simulink model "Sano"  (R2024b)
settings: Solver=ode15s  StartTime=0.0  StopTime=30.0  MaxStep=1E-3  RelTol=1e-3
libraries: slpidlib x1
settings Model: Creator=leslie  LastModifiedBy=leslie
settings DataIOCC: ReturnWorkspaceOutputs=off  TimeSaveName=t
settings DebuggingCC: AlgebraicLoopMsg=none  ArtificialAlgebraicLoopMsg=none  MaxConsecutiveZCsMsg=none  InheritedTsInSrcMsg=none  MultiTaskCondExecSysMsg=none  UnknownTsInhSupMsg=none  OperatingPointInterfaceChecksumMismatchMsg=none

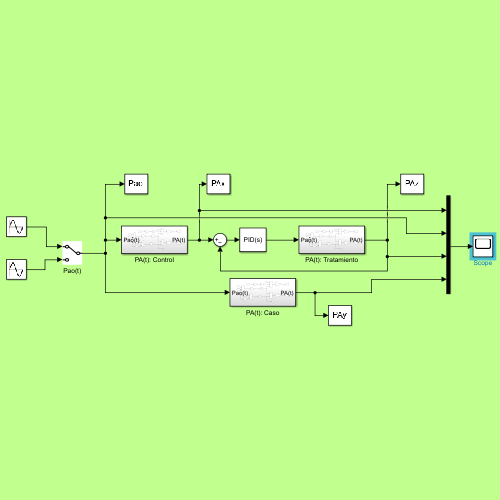
[thumbnail: Simulink's stored preview of the top-level diagram]
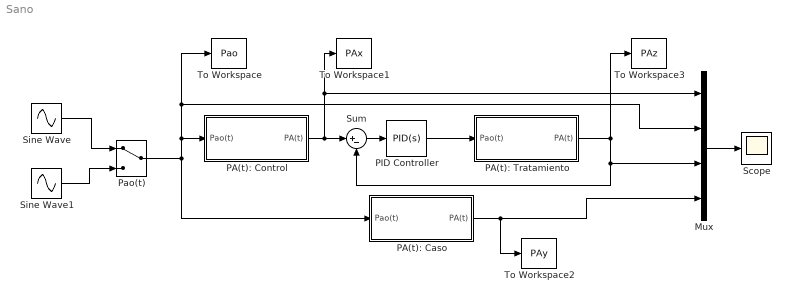
== system Sano ==
  Mux : Mux
  PA(t): Caso : Subsystem
  PA(t): Control : Subsystem
  PA(t): Tratamiento : Subsystem
  PID Controller : slpidlib/PID Controller  Controller=PID  Form=Parallel  TimeDomain=Continuous-time  UseExternalTs=off  SampleTime=-1  IntegratorMethod=Forward Euler  FilterMethod=Forward Euler  ControllerParametersSource=internal  P=15.8953606940144  I=452.120770004536  UseKiTs=off  D=0.0428965162903509  UseExternalDerivativeSource=off  N=198.651405283432  UseFilter=on  TunerSelectOption=Transfer Function Based (PID Tuner App)  InitialConditionSource=internal  InitialConditionForIntegrator=0  InitialConditionForFilter=0  DifferentiatorICPrevScaledInput=0  ExternalReset=none  TrackingMode=off  Kt=1  LimitOutput=off  SatLimitsSource=internal  UpperSaturationLimit=inf  LowerSaturationLimit=-inf  LinearizeAsGain=on  AntiWindupMode=none  Kb=1  LimitIntegrator=off  UpperIntegratorSaturationLimit=inf  LowerIntegratorSaturationLimit=-inf  POutMin=[]  POutMax=[]  IOutMin=[]  IOutMax=[]  DOutMin=[]  DOutMax=[]  NOutMin=[]  NOutMax=[]  SumOutMin=[]  SumOutMax=[]  SaturationOutMin=[]  SaturationOutMax=[]  PParamMin=[]  PParamMax=[]  IParamMin=[]  IParamMax=[]  DParamMin=[]  DParamMax=[]  NParamMin=[]  NParamMax=[]  KbParamMin=[]  KbParamMax=[]  KtParamMin=[]  KtParamMax=[]  KbOutMin=[]  KbOutMax=[]  KtOutMin=[]  KtOutMax=[]  IntegratorOutMin=[]  IntegratorOutMax=[]  FilterOutMin=[]  FilterOutMax=[]  SumI1OutMin=[]  SumI1OutMax=[]  SumI2OutMin=[]  SumI2OutMax=[]  SumI3OutMin=[]  SumI3OutMax=[]  SumI4OutMin=[]  SumI4OutMax=[]  SumDOutMin=[]  SumDOutMax=[]  DifferentiatorOutMin=[]  DifferentiatorOutMax=[]  FilterDiffOutCoefMin=[]  FilterDiffOutCoefMax=[]  ReciprocalOutMin=[]  ReciprocalOutMax=[]  SumDenOutMin=[]  SumDenOutMax=[]  SumNumOutMin=[]  SumNumOutMax=[]  DivideOutMin=[]  DivideOutMax=[]  UdiffTsProdOutMin=[]  UdiffTsProdOutMax=[]  NTsProdOutMin=[]  NTsProdOutMax=[]  UintegralTsProdOutMin=[]  UintegralTsProdOutMax=[]  UngainTsProdOutMin=[]  UngainTsProdOutMax=[]  ClampingZeroOutDataTypeStr=Inherit: Inherit via back propagation  ClampingZeroOutMin=[]  ClampingZeroOutMax=[]  FilterDenConstantOutDataTypeStr=Inherit: Inherit via back propagation  FilterDenConstantOutMin=[]  FilterDenConstantOutMax=[]  PCopyOutDataTypeStr=Inherit: Inherit via back propagation  PCopyOutMin=[]  PCopyOutMax=[]  NCopyOutDataTypeStr=Inherit: Inherit via back propagation  NCopyOutMin=[]  NCopyOutMax=[]  IntegratorContinuousStateAttributes=''  IntegratorStateMustResolveToSignalObject=off  IntegratorRTWStateStorageClass=Auto  FilterContinuousStateAttributes=''  FilterStateMustResolveToSignalObject=off  FilterRTWStateStorageClass=Auto  ParallelPVariant=InternalParameters  IdealPVariant=Disabled  IVariant=InternalParameters  DVariant=InternalParameters  IntegratorVariant=Continuous  SatVariant=Disabled  AWVariant=Passthrough  PCopyVariant=Disabled  TRVariant=Disabled  FdbkBlocksVariant=Forward  IdealPFdbkVariant=Disabled  SatFdbkVariant=Disabled  DerivativeFilterVariant=ContFilter  NVariant=InternalParameters  NCopyVariant=Disabled  FilterICVariant=InternalICsFilter  IntegratorICVariant=InternalICs  ExternalResetVariant=Disabled  TRSumVariant=Passthrough  SumFdbkVariant=Disabled  SumVariant=Sum_PID  TsampFilterVariant=InternalTs  TsampNgainVariant=Passthrough  TsampIntegralVariant=Disabled_SignalSpec  ExternalSaturationOutDataTypeStr=Inherit: Same as second input  DerivativeSourceVariant=ErrorSignal  PreIntVariant=InternalPreInt
  Pao(t) : ManualSwitch
  Scope : Scope
  Sine Wave : Sin  Amplitude=2.5  Frequency=1.5708  SampleTime=0
  Sine Wave1 : Sin  Amplitude=2.5  Frequency=2*pi*500E-3  SampleTime=0
  Sum : Sum  Inputs=|+-
  To Workspace : ToWorkspace  VariableName=Pao  SampleTime=-1
  To Workspace1 : ToWorkspace  VariableName=PAx  SampleTime=-1
  To Workspace2 : ToWorkspace  VariableName=PAy  SampleTime=-1
  To Workspace3 : ToWorkspace  VariableName=PAz  SampleTime=-1
  wires:
  Sum/1 -> PID Controller/1
  Pao(t)/1 -> PA(t): Caso/1(Pao(t)), PA(t): Control/1(Pao(t)), To Workspace/1, Mux/2
  Sine Wave/1 -> Pao(t)/1
  Sine Wave1/1 -> Pao(t)/2
  Mux/1 -> Scope/1
  PA(t): Caso/1(PA(t)) -> To Workspace2/1, Mux/4
  PID Controller/1 -> PA(t): Tratamiento/1(Pao(t))
  PA(t): Tratamiento/1(PA(t)) -> Mux/3, Sum/2, To Workspace3/1
  PA(t): Control/1(PA(t)) -> Sum/1, Mux/1, To Workspace1/1

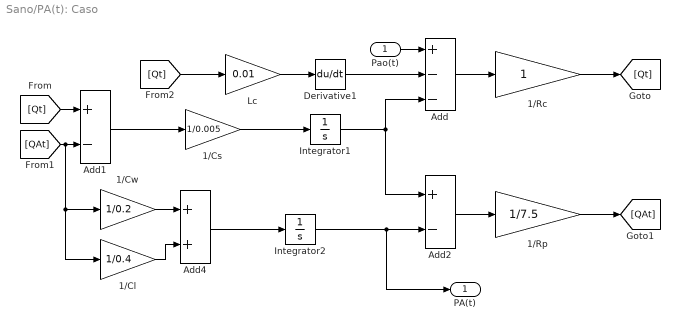
== system Sano/PA(t): Caso ==
  Pao(t) : Inport
  1/Cl : Gain  Gain=1/0.4
  1/Cs : Gain  Gain=1/0.005
  1/Cw : Gain  Gain=1/0.2
  1/Rc : Gain
  1/Rp : Gain  Gain=1/7.5
  Add : Sum  Inputs=+--
  Add1 : Sum  Inputs=+-
  Add2 : Sum  Inputs=+-
  Add4 : Sum
  Derivative1 : Derivative
  Integrator1 : Integrator
  Integrator2 : Integrator
  Lc : Gain  Gain=0.01
  PA(t) : Outport
  wires:
  1/Cw/1 -> Add4/1
  Derivative1/1 -> Add/2
  1/Cs/1 -> Integrator1/1
  Integrator1/1 -> Add2/1, Add/3
  [Qt] -> Lc/1
  Integrator2/1 -> PA(t)/1, Add2/2
  Lc/1 -> Derivative1/1
  Add4/1 -> Integrator2/1
  1/Rc/1 -> [Qt]
  Pao(t)/1 -> Add/1
  Add2/1 -> 1/Rp/1
  Add/1 -> 1/Rc/1
  [QAt] -> 1/Cl/1, 1/Cw/1, Add1/2
  Add1/1 -> 1/Cs/1
  [Qt] -> Add1/1
  1/Rp/1 -> [QAt]
  1/Cl/1 -> Add4/2

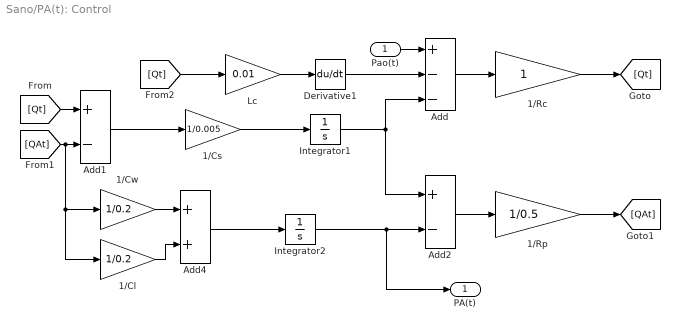
== system Sano/PA(t): Control ==
  Pao(t) : Inport
  1/Cl : Gain  Gain=1/0.2
  1/Cs : Gain  Gain=1/0.005
  1/Cw : Gain  Gain=1/0.2
  1/Rc : Gain
  1/Rp : Gain  Gain=1/0.5
  Add : Sum  Inputs=+--
  Add1 : Sum  Inputs=+-
  Add2 : Sum  Inputs=+-
  Add4 : Sum
  Derivative1 : Derivative
  Integrator1 : Integrator
  Integrator2 : Integrator
  Lc : Gain  Gain=0.01
  PA(t) : Outport
  wires:
  Pao(t)/1 -> Add/1
  Add/1 -> 1/Rc/1
  [Qt] -> Add1/1
  [QAt] -> 1/Cl/1, 1/Cw/1, Add1/2
  1/Rc/1 -> [Qt]
  Add2/1 -> 1/Rp/1
  1/Rp/1 -> [QAt]
  Derivative1/1 -> Add/2
  [Qt] -> Lc/1
  Lc/1 -> Derivative1/1
  Integrator1/1 -> Add2/1, Add/3
  1/Cs/1 -> Integrator1/1
  Add1/1 -> 1/Cs/1
  Integrator2/1 -> PA(t)/1, Add2/2
  1/Cw/1 -> Add4/1
  1/Cl/1 -> Add4/2
  Add4/1 -> Integrator2/1

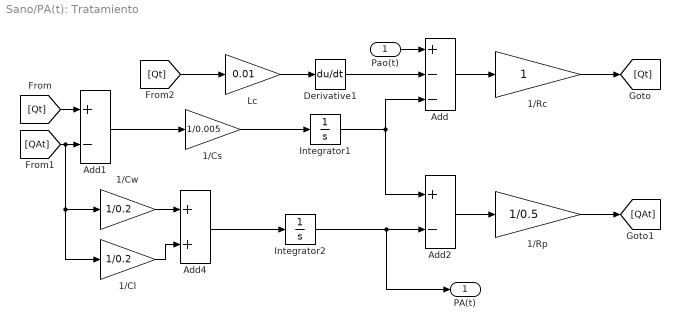
== system Sano/PA(t): Tratamiento ==
  Pao(t) : Inport
  1/Cl : Gain  Gain=1/0.2
  1/Cs : Gain  Gain=1/0.005
  1/Cw : Gain  Gain=1/0.2
  1/Rc : Gain
  1/Rp : Gain  Gain=1/0.5
  Add : Sum  Inputs=+--
  Add1 : Sum  Inputs=+-
  Add2 : Sum  Inputs=+-
  Add4 : Sum
  Derivative1 : Derivative
  Integrator1 : Integrator
  Integrator2 : Integrator
  Lc : Gain  Gain=0.01
  PA(t) : Outport
  wires:
  1/Cw/1 -> Add4/1
  Derivative1/1 -> Add/2
  1/Cs/1 -> Integrator1/1
  Integrator1/1 -> Add2/1, Add/3
  [Qt] -> Lc/1
  Integrator2/1 -> PA(t)/1, Add2/2
  Lc/1 -> Derivative1/1
  Add4/1 -> Integrator2/1
  1/Rc/1 -> [Qt]
  Pao(t)/1 -> Add/1
  Add2/1 -> 1/Rp/1
  Add/1 -> 1/Rc/1
  [QAt] -> 1/Cl/1, 1/Cw/1, Add1/2
  Add1/1 -> 1/Cs/1
  [Qt] -> Add1/1
  1/Rp/1 -> [QAt]
  1/Cl/1 -> Add4/2
